simulink model "HRXDUAL_Delay"  (R2023b)
settings: Solver=FixedStepDiscrete  StartTime=0.0  StopTime=Inf  FixedStep=0.0001  RelTol=1e-3  EnableMultiTasking=on
libraries: canmsglib x24, c280xlib x24, simulink x11
(part 2 of 2)

== system HRXDUAL_Delay/Read position2/Subsystem5/Delay 1ms4/System Outputs ==

== system HRXDUAL_Delay/Read position2/Subsystem5/Delay 1ms5/System Outputs ==

== system HRXDUAL_Delay/Read position2/Subsystem5/Delay 1ms6/System Outputs ==

== system HRXDUAL_Delay/Read position2/Subsystem5/Delay 1ms7/System Outputs ==

== system HRXDUAL_Delay/Read position2/Subsystem5/Delay 1ms8/System Outputs ==

== system HRXDUAL_Delay/Read position2/Subsystem5/Delay 1ms9/System Outputs ==

== matlab function HRXDUAL_Delay/MATLAB Function ==
  data: torque1int output; joKd input; pos1 input; vel1 input
function torque1int  = computeRobTorques(joKd, pos1, vel1)

    % This function computes the output torque to apply to the robot as a
    % function of the control mode and of human-human connection gains.
    % Inputs:
    %    - joKd    : 1x1 float: Joint viscosity
    %    - pos1    : 1x1 float: Current position of robot 1 [rad]
    %    - vel1    : 1x1 float: Current velocity of robot 1 [rad/s]
    % Outputs:
    %    - torque1: 1x1 int: Current torque order for robot 1 [mNm]
    

    % Adjust angles to align offsets
    pos1 = pos1 + 1.994;

    % only robot joint viscosity damping
    torque1 = -joKd * vel1;


    % Transorm torques to integers
    torque1int = fix(1000 * torque1);
end
